simulink model "PID_sim"  (R2022b)
settings: Solver=VariableStepAuto  StartTime=0.0  StopTime=5  FixedStep=0.001  RelTol=1e-3
libraries: cstblocks x2
settings Model: Creator=jprivera  LastModifiedBy=jprivera

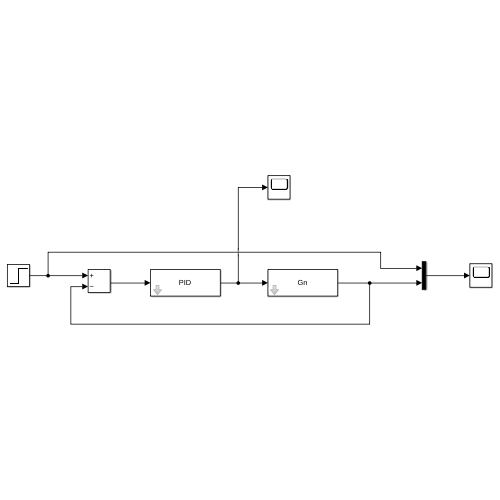
[thumbnail: Simulink's stored preview of the top-level diagram]
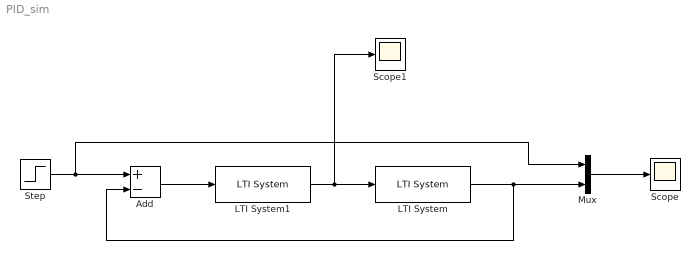
== system PID_sim ==
  Add : Sum  Inputs=+-
  LTI System : cstblocks/LTI System  sys=Gn  IC=[]
  LTI System1 : cstblocks/LTI System  sys=PID  IC=[]
  Mux : Mux  Inputs=2
  Scope : Scope
  Scope1 : Scope
  Step : Step  SampleTime=0
  wires:
  LTI System1/1 -> Scope1/1, LTI System/1
  LTI System/1 -> Add/2, Mux/2
  Mux/1 -> Scope/1
  Add/1 -> LTI System1/1
  Step/1 -> Mux/1, Add/1
